simulink model "Motor_Step_Response_Linear_1st_2nd_Coulomb"  (R2016b)
settings: Solver=ode5  StartTime=0.0  StopTime=Tsim_final  FixedStep=sim_step_size  RelTol=1e-3
undefined symbols (not defined in the file): Bm, Jm, Kb, Kt, Lm, Rm, Vsupply
settings Model: Creator=Mac  LastModifiedBy=Mac

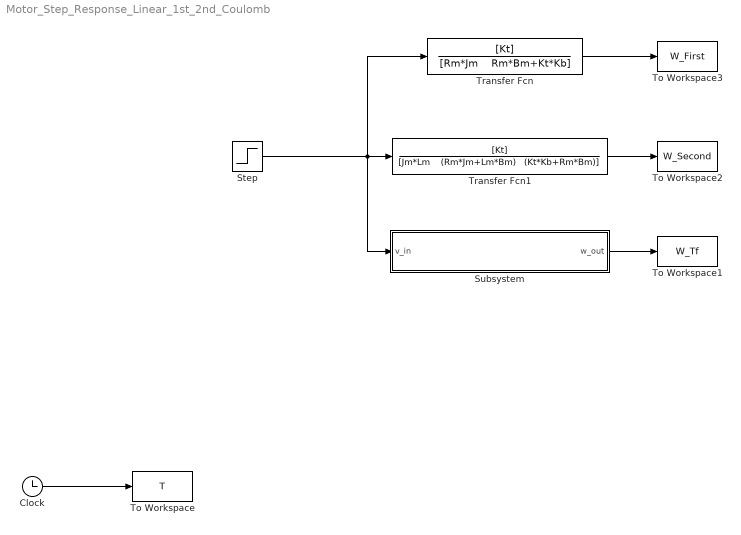
== system Motor_Step_Response_Linear_1st_2nd_Coulomb ==
  Clock : Clock
  Step : Step  Time=0  After=Vsupply  SampleTime=0
  Subsystem : Subsystem
  To Workspace : ToWorkspace  VariableName=T  SampleTime=-1
  To Workspace1 : ToWorkspace  VariableName=W_Tf  SampleTime=-1
  To Workspace2 : ToWorkspace  VariableName=W_Second  SampleTime=-1
  To Workspace3 : ToWorkspace  VariableName=W_First  SampleTime=-1
  Transfer Fcn : TransferFcn  Numerator=[Kt]  Denominator="[Rm*Jm    Rm*Bm+Kt*Kb]"
  Transfer Fcn1 : TransferFcn  Numerator=[Kt]  Denominator="[Jm*Lm    (Rm*Jm+Lm*Bm)   (Kt*Kb+Rm*Bm)]"
  wires:
  Clock/1 -> To Workspace/1
  Transfer Fcn/1 -> To Workspace3/1
  Transfer Fcn1/1 -> To Workspace2/1
  Subsystem/1(w_out) -> To Workspace1/1
  Step/1 -> Subsystem/1(v_in), Transfer Fcn1/1, Transfer Fcn/1

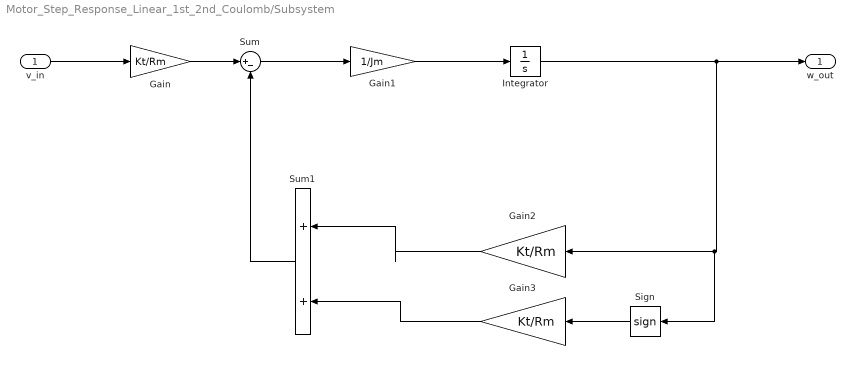
== system Motor_Step_Response_Linear_1st_2nd_Coulomb/Subsystem ==
  v_in : Inport
  Gain : Gain  Gain=Kt/Rm
  Gain1 : Gain  Gain=1/Jm
  Gain2 : Gain  Gain=Kt/Rm
  Gain3 : Gain  Gain=Kt/Rm
  Integrator : Integrator
  Sign : Signum
  Sum : Sum  Inputs=|+-
  Sum1 : Sum  Inputs=|++
  w_out : Outport
  wires:
  Integrator/1 -> Sign/1, Gain2/1, w_out/1
  Gain1/1 -> Integrator/1
  Sum/1 -> Gain1/1
  Gain/1 -> Sum/1
  Sum1/1 -> Sum/2
  Gain2/1 -> Sum1/1
  Gain3/1 -> Sum1/2
  Sign/1 -> Gain3/1
  v_in/1 -> Gain/1
